simulink library "motorAndLoadSimPowerSystemsLib"  (R2019a)
settings: Solver=ode45  StartTime=0.0  StopTime=10.0  RelTol=1e-3  EnableMultiTasking=on
undefined symbols (not defined in the file): adc, encoder, inverter, pmsm, pwm
libraries: fl_lib x26, nesl_utility x16, ee_lib x6
settings Model: Creator=The MathWorks, Inc.  LastModifiedBy=The MathWorks, Inc.
settings DataIOCC: LimitDataPoints=on  SaveFormat=Array  ReturnWorkspaceOutputs=off
settings OptimizationCC: ExpressionDepthLimit=2147483647  LifeSpan=inf
settings DebuggingCC: UnderspecifiedInitializationDetection=Classic  MergeDetectMultiDrivingBlocksExec=none  SolverPrmCheckMsg=warning  AllowSymbolicDim=off  StateNameClashWarn=warning  SFUnexpectedBacktrackingDiag=warning  SFNoUnconditionalDefaultTransitionDiag=warning  SFExecutionAtInitializationDiag=none  ArithmeticOperatorsInVariantConditions=warning
settings HardwareCC: ProdBitPerPointer=32  ProdBitPerSizeT=32  ProdBitPerPtrDiffT=32  ProdLargestAtomicFloat=None  ProdIntDivRoundTo=Undefined  ProdEndianess=Unspecified  ProdWordSize=32  ProdHWDeviceType=32-bit Generic
settings ModelReferenceCC: PropagateSignalLabelsOutOfModel=off
settings SFSimCC: SimUseLocalCustomCode=off
settings RTWCC: RTWUseLocalCustomCode=off
settings CodeAppCC: StateflowObjectComments=on
settings GRTTargetCC: TargetLangStandard=C89/C90 (ANSI)  GeneratePreprocessorConditionals=Disable all
settings ConfigComp: CovMetricSettings=dw  CovHtmlReporting=on  CovSaveCumulativeToWorkspaceVar=on  CovSaveSingleToWorkspaceVar=on  CovExternalEMLEnable=off  CovSFcnEnable=off

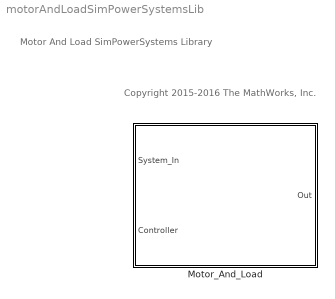
== system motorAndLoadSimPowerSystemsLib ==
  note: Motor And Load SimPowerSystems Library
  note: Copyright 2015-2016 The MathWorks, Inc.
  Motor_And_Load : Subsystem
      mask Display: image('focZynqMotorAndLoadMask.png');

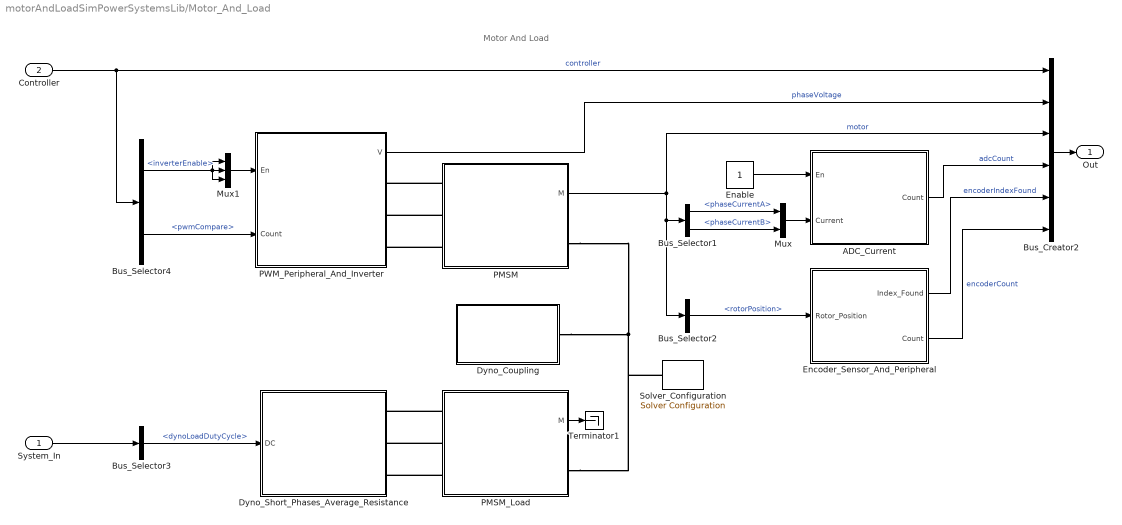
== system motorAndLoadSimPowerSystemsLib/Motor_And_Load ==
  note: Motor And Load
  System_In : Inport
  Controller : Inport  Port=2
  ADC_Current : Subsystem
      mask Display:
      | image('adcCurrentMask.png')
      | port_label('input',1,'En')
      | port_label('input',2,'I')
      | port_label('output',1,'Count')
  Bus_Creator2 : BusCreator  Inputs=6
  Bus_Selector1 : BusSelector  OutputSignals=phaseCurrentA,phaseCurrentB
  Bus_Selector2 : BusSelector  OutputSignals=rotorPosition
  Bus_Selector3 : BusSelector  OutputSignals=dynoLoadDutyCycle
  Bus_Selector4 : BusSelector  OutputSignals=inverterEnable,pwmCompare
  Dyno_Coupling : Subsystem  VariantControl=loadType == motorLoad.disc
      mask Display: image('dynoCouplingMask.png')
  Dyno_Short_Phases_Average_Resistance : Subsystem
      mask Display:
      | image('dynoShortPhasesAverageResistance.png')
      | text(0.03, 0.50, 'DC', 'HorizontalAlignment', 'Left')
      | text(0.98, 0.80, 'A',  'HorizontalAlignment', 'Right')
      | text(0.98, 0.50, 'B',  'HorizontalAlignment', 'Right')
      | text(0.98, 0.20, 'C',  'HorizontalAlignment', 'Right')
  Enable : Constant  SampleTime=-1
  Encoder_Sensor_And_Peripheral : Subsystem
      mask Display:
      | image('encoderSensorAndPeripheralMask.png')
      | port_label('input',1,'P')
      | port_label('output',1,sprintf('Index\nFound')')
      | port_label('output',2,'Count')
  Mux : Mux  Inputs=2
  Mux1 : Mux  Inputs=3
  PMSM : Subsystem
      mask Display:
      | image('pmsmMask.png')
      | text(0.03, 0.80, 'A', 'HorizontalAlignment', 'Left')
      | text(0.03, 0.50, 'B', 'HorizontalAlignment', 'Left')
      | text(0.03, 0.20, 'C', 'HorizontalAlignment', 'Left')
      | text(0.98, 0.75, 'M', 'HorizontalAlignment', 'Right')
      | text(0.98, 0.25, 'R', 'HorizontalAlignment', 'Right')
  PMSM_Load : Subsystem
      mask Display:
      | image('pmsmMask.png')
      | text(0.03, 0.80, 'A', 'HorizontalAlignment', 'Left')
      | text(0.03, 0.50, 'B', 'HorizontalAlignment', 'Left')
      | text(0.03, 0.20, 'C', 'HorizontalAlignment', 'Left')
      | text(0.98, 0.75, 'M', 'HorizontalAlignment', 'Right')
      | text(0.98, 0.25, 'R', 'HorizontalAlignment', 'Right')
  PWM_Peripheral_And_Inverter : Subsystem  VariantControl=variantPwm == enumPwm.behavior
      mask Display:
      | image('pwmPeripheralAndInverterMask.png')
      | port_label('output',1,'V')
      | port_label('input',1,'En')
      | port_label('input',2,'Compare')
      | text(0.98, 0.64, 'A', 'HorizontalAlignment', 'Right')
      | text(0.98, 0.38, 'B', 'HorizontalAlignment', 'Right')
      | text(0.98, 0.12, 'C', 'HorizontalAlignment', 'Right')
  Solver_Configuration : nesl_utility/Solver Configuration  PhysicalDomain=network_engine_domain  SubClassName=solver  LeftPortType=input  RightPortType=generic  Tones=[]  Harmonics=[]  SimulateNoise=off  Profile=off  UseLocalSampling=off  EnableSwitchedLinearOptims=on  FrequencyDomain=off  UseCCode=off  RelTol=0.001  AbsTol=1e-06  MinStep=1e-09  ToWorkspace=off  RevertToSquareIcSolve=off  NumHomotopyIterations=100  PhasorMode=off  PhasorModeNumHarmonics=1  DoDC=off  ResidualTolerance=1e-9  UseLocalSolver=on  LocalSolverChoice=NE_BACKWARD_EULER_ADVANCER  LocalSolverSampleTime=40e-6  DoFixedCost=on  MaxNonlinIter=3  MaxModeIter=2  LinearAlgebra=Sparse  EquationFormulation=NE_TIME_EF  DelaysMemoryBudget=1024  AutomaticFiltering=on  FilteringTimeConstant=0.001  PartitionStorageMethod=AS_NEEDED  PartitionMemoryBudget=1024  PartitionMethod=FAST
  Terminator1 : Terminator
  Out : Outport
  wires:
  Mux1/1 -> PWM_Peripheral_And_Inverter/1(En)
  Bus_Selector3/1 -> Dyno_Short_Phases_Average_Resistance/1(DC)  "<dynoLoadDutyCycle>"
  PMSM_Load/1(M) -> Terminator1/1
  PWM_Peripheral_And_Inverter/1(V) -> Bus_Creator2/2  "phaseVoltage"
  System_In/1 -> Bus_Selector3/1
  Encoder_Sensor_And_Peripheral/2(Count) -> Bus_Creator2/6  "encoderCount"
  Encoder_Sensor_And_Peripheral/1(Index_Found) -> Bus_Creator2/5  "encoderIndexFound"
  ADC_Current/1(Count) -> Bus_Creator2/4  "adcCount"
  Bus_Selector4/2 -> PWM_Peripheral_And_Inverter/2(Count)  "<pwmCompare>"
  Bus_Selector4/1 -> Mux1/2, Mux1/3, Mux1/1  "<inverterEnable>"
  Bus_Selector2/1 -> Encoder_Sensor_And_Peripheral/1(Rotor_Position)  "<rotorPosition>"
  Mux/1 -> ADC_Current/2(Current)
  Bus_Selector1/2 -> Mux/2  "<phaseCurrentB>"
  Bus_Selector1/1 -> Mux/1  "<phaseCurrentA>"
  Controller/1 -> Bus_Creator2/1, Bus_Selector4/1  "controller"
  Bus_Creator2/1 -> Out/1
  PMSM/1(M) -> Bus_Selector2/1, Bus_Selector1/1, Bus_Creator2/3  "motor"
  Enable/1 -> ADC_Current/1(En)
  connections:
  PMSM_Load/LConn3 -- Dyno_Short_Phases_Average_Resistance/RConn3
  PMSM_Load/LConn2 -- Dyno_Short_Phases_Average_Resistance/RConn2
  PMSM_Load/LConn1 -- Dyno_Short_Phases_Average_Resistance/RConn1
  PMSM/RConn1 -- Dyno_Coupling/RConn1 -- PMSM_Load/RConn1 -- Solver_Configuration/RConn1
  PMSM/LConn1 -- PWM_Peripheral_And_Inverter/RConn1
  PMSM/LConn2 -- PWM_Peripheral_And_Inverter/RConn2
  PMSM/LConn3 -- PWM_Peripheral_And_Inverter/RConn3

== system motorAndLoadSimPowerSystemsLib/Motor_And_Load/ADC_Current ==
  note: ADC Current
  En : Inport
  Current : Inport  Port=2
  ADC : Subsystem
      mask Display:
      | image('adcMask.png')
      | port_label('input',1,'V_T','texmode', 'on')
      | port_label('output',1,'Count')
  Current_Transducer : Subsystem
      mask Display:
      | image('currentTransducerMask.png')
      | port_label('input', 1,'En')
      | port_label('input', 2,'I')
      | port_label('output',1,'V_T','texmode', 'on')
  Count : Outport
  wires:
  Current/1 -> Current_Transducer/2(Current)
  En/1 -> Current_Transducer/1(En)
  Current_Transducer/1(V_T) -> ADC/1(Volt)  "transducerVoltage"
  ADC/1(Count) -> Count/1

== system motorAndLoadSimPowerSystemsLib/Motor_And_Load/Dyno_Coupling ==
  note: Dyno Coupling
  Inertia : fl_lib/Mechanical/Rotational Elements/Inertia  inertia=dynoCoupling.Inertia kg*m^2  w_specify=on  w_priority=High  w=pmsm.RotorVelocityInit rad/s  w_nominal_specify=off  w_nominal_unit=rad/s  w_nominal_value=1  t_specify=off  t_priority=High  t=0 N*m  t_nominal_specify=off  t_nominal_unit=N*m  t_nominal_value=1
      settings: AttributesFormatString=|
      | ---------------------------------------
      | Inertia = %<inertia>
  R : PMIOPort  Side=Right
  connections:
  Inertia/LConn1 -- R/RConn1

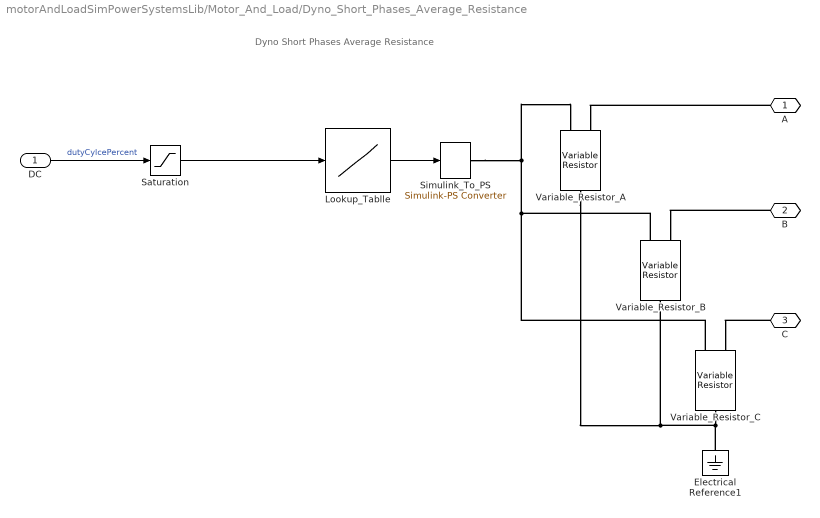
== system motorAndLoadSimPowerSystemsLib/Motor_And_Load/Dyno_Short_Phases_Average_Resistance ==
  note: Dyno Short Phases Average Resistance
  DC : Inport
  Electrical Reference1 : fl_lib/Electrical/Electrical Elements/Electrical Reference
  Lookup_Tablle : Lookup_n-D  NumberOfTableDimensions=1  BreakpointsForDimension1=[0 10 20 30 40 50 60 70 80 90 95 100]  Table=[2000 800 250 130 60 40 28 21 15 2.3 1.03 0]  ExtrapMethod=Clip  InternalRulePriority=Speed  RndMeth=Simplest  InputSameDT=on
      settings: AttributesFormatString=|
      | -----------------------------------------------------------------------
      | DutyCycle = %<BreakpointsForDimension1>
      | Resistance = %<Table>
  Saturation : Saturate  UpperLimit=100  LowerLimit=0
      settings: AttributesFormatString=|
      | ------------------------------
      | UpperLimit = %<UpperLimit>
      | LowerLimit = %<LowerLimit>
  Simulink_To_PS : nesl_utility/Simulink-PS Converter  PhysicalDomain=network_engine_domain  SubClassName=ps_input  LeftPortType=input  RightPortType=output  PseudoPeriodic=off  Frequencies=[]  NoiseDistribution=none  NoiseParameters=[]  Unit=1  AffineConversion=off  FilteringAndDerivatives=filter  SimscapeFilterOrder=1  InputFilterTimeConstant=0.001  UdotUserProvided=1
  Variable_Resistor_A : fl_lib/Electrical/Electrical Elements/Variable Resistor  Rmin=0 Ohm  i_specify=off  i_priority=None  i=0 A  i_nominal_specify=off  i_nominal_unit=A  i_nominal_value=1  v_specify=off  v_priority=None  v=0 V  v_nominal_specify=off  v_nominal_unit=V  v_nominal_value=1
  Variable_Resistor_B : fl_lib/Electrical/Electrical Elements/Variable Resistor  Rmin=0 Ohm  i_specify=off  i_priority=None  i=0 A  i_nominal_specify=off  i_nominal_unit=A  i_nominal_value=1  v_specify=off  v_priority=None  v=0 V  v_nominal_specify=off  v_nominal_unit=V  v_nominal_value=1
  Variable_Resistor_C : fl_lib/Electrical/Electrical Elements/Variable Resistor  Rmin=0 Ohm  i_specify=off  i_priority=None  i=0 A  i_nominal_specify=off  i_nominal_unit=A  i_nominal_value=1  v_specify=off  v_priority=None  v=0 V  v_nominal_specify=off  v_nominal_unit=V  v_nominal_value=1
  A : PMIOPort  Side=Right
  B : PMIOPort  Port=2  Side=Right
  C : PMIOPort  Port=3  Side=Right
  wires:
  Lookup_Tablle/1 -> Simulink_To_PS/1
  Saturation/1 -> Lookup_Tablle/1
  DC/1 -> Saturation/1  "dutyCylcePercent"
  connections:
  B/RConn1 -- Variable_Resistor_B/LConn2
  C/RConn1 -- Variable_Resistor_C/LConn2
  Variable_Resistor_C/RConn1 -- Electrical Reference1/LConn1 -- Variable_Resistor_A/RConn1 -- Variable_Resistor_B/RConn1
  A/RConn1 -- Variable_Resistor_A/LConn2
  Variable_Resistor_B/LConn1 -- Variable_Resistor_C/LConn1 -- Simulink_To_PS/RConn1 -- Variable_Resistor_A/LConn1

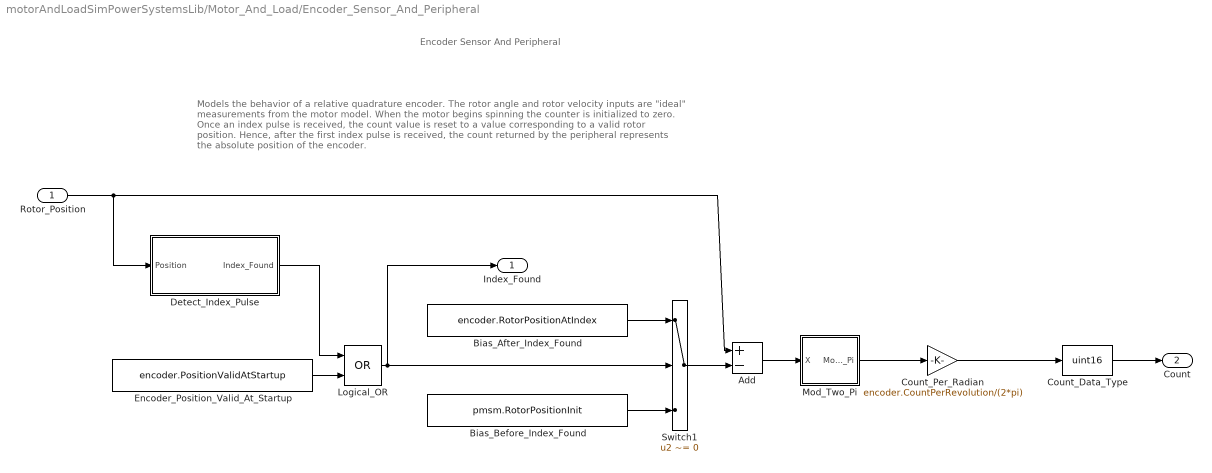
== system motorAndLoadSimPowerSystemsLib/Motor_And_Load/Encoder_Sensor_And_Peripheral ==
  note: Models the behavior of a relative quadrature encoder. The rotor angle and rotor velocity inputs are "ideal" measurements from the motor model.
      | When the motor begins spinning the counter is initialized to zero.
      | Once an index pulse is received, the count value is reset to a value corresponding to a valid rotor position.
      | Hence, after the first index pulse is received, the count returned by the peripheral represents the absolute position of the encoder.
  note: Encoder Sensor And Peripheral
  Rotor_Position : Inport
  Add : Sum  Inputs=+-
  Bias_After_Index_Found : Constant  Value=encoder.RotorPositionAtIndex
  Bias_Before_Index_Found : Constant  Value=pmsm.RotorPositionInit
  Count_Data_Type : DataTypeConversion  OutDataTypeStr=uint16
  Count_Per_Radian : Gain  Gain=encoder.CountPerRevolution/(2*pi)
      settings: AttributesFormatString=|
      | ------------------------------------------
      | Gain = %<Gain>
  Detect_Index_Pulse : Subsystem
  Encoder_Position_Valid_At_Startup : Constant  Value=encoder.PositionValidAtStartup
  Logical_OR : Logic  Operator=OR  IconShape=distinctive  AllPortsSameDT=off  OutDataTypeStr=boolean
  Mod_Two_Pi : Subsystem
      mask Display:
      | text(0.5, 0.5,'Mod 2\pi',...
      |   'HorizontalAlignment', 'Center',...
      |   'VerticalAlignment', 'Middle',...
      |   'texmode', 'on')
  Switch1 : Switch  Criteria=u2 ~= 0
  Index_Found : Outport
  Count : Outport  Port=2
  wires:
  Bias_Before_Index_Found/1 -> Switch1/3
  Bias_After_Index_Found/1 -> Switch1/1
  Logical_OR/1 -> Index_Found/1, Switch1/2
  Encoder_Position_Valid_At_Startup/1 -> Logical_OR/2
  Detect_Index_Pulse/1(Index_Found) -> Logical_OR/1
  Rotor_Position/1 -> Add/1, Detect_Index_Pulse/1(Position)
  Mod_Two_Pi/1(Mod_X_Two_Pi) -> Count_Per_Radian/1
  Count_Data_Type/1 -> Count/1
  Switch1/1 -> Add/2
  Add/1 -> Mod_Two_Pi/1(X)
  Count_Per_Radian/1 -> Count_Data_Type/1

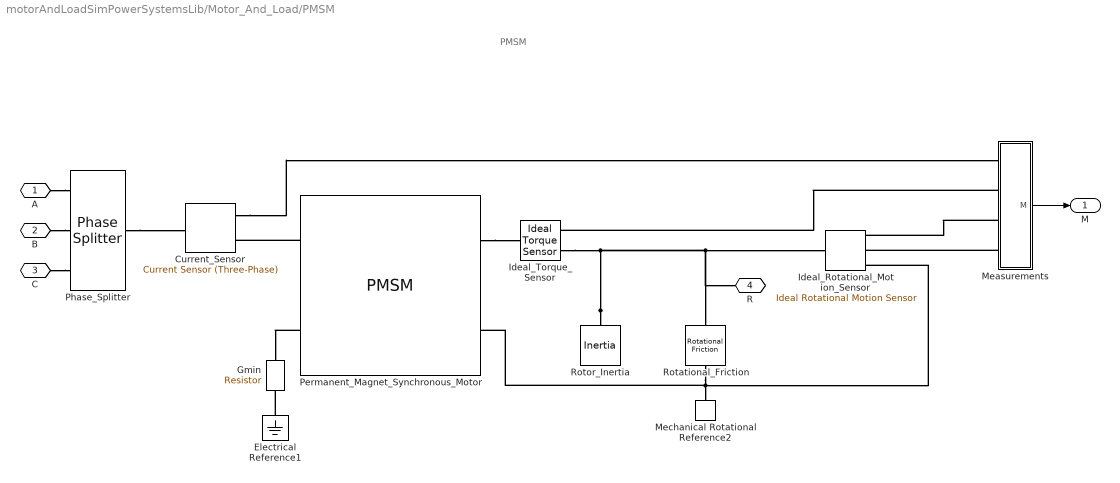
== system motorAndLoadSimPowerSystemsLib/Motor_And_Load/PMSM ==
  note: PMSM
  Current_Sensor : ee_lib/Sensors & Transducers/Current Sensor (Three-Phase)
      settings: SourceProductName=Simscape Electrical
  Electrical Reference1 : fl_lib/Electrical/Electrical Elements/Electrical Reference
  Gmin : fl_lib/Electrical/Electrical Elements/Resistor  R=1e9 Ohm  i_specify=off  i_priority=None  i=0 A  i_nominal_specify=off  i_nominal_unit=A  i_nominal_value=1  v_specify=off  v_priority=None  v=0 V  v_nominal_specify=off  v_nominal_unit=V  v_nominal_value=1
  Ideal_Rotational_Mot ion_Sensor : fl_lib/Mechanical/Mechanical Sensors/Ideal Rotational Motion Sensor  offset=pmsm.RotorPositionInit rad
  Ideal_Torque_Sensor : fl_lib/Mechanical/Mechanical Sensors/Ideal Torque Sensor
  Measurements : Subsystem
  Mechanical Rotational Reference2 : fl_lib/Mechanical/Rotational Elements/Mechanical Rotational Reference
  Permanent_Magnet_Synchronous_Motor : ee_lib/Electromechanical/Permanent Magnet/PMSM  nPolePairs=pmsm.PolePairs  pmflux_param=1  pm_flux_linkage=pmsm.FluxLinkage Wb  torque_constant=0.18 N*m/A  back_emf_constant=0.18 V/(rad/s)  stator_param=1  Ld=pmsm.InductanceLd H  Lq=pmsm.InductanceLq H  L0=pmsm.InductanceL0 H  Ls=0.0002 H  Lm=0 H  Ms=0 H  Rs=pmsm.StatorPhaseResistance Ohm  zero_sequence=ee.enum.park.zerosequence.include  J=0 kg*m^2  lam=0 N*m/(rad/s)  axes_param=2  i_d_specify=off  i_d_priority=None  i_d=0 A  i_d_nominal_specify=off  i_d_nominal_unit=A  i_d_nominal_value=1  i_q_specify=off  i_q_priority=None  i_q=0 A  i_q_nominal_specify=off  i_q_nominal_unit=A  i_q_nominal_value=1  torque_specify=off  torque_priority=None  torque=0 N*m  torque_nominal_specify=off  torque_nominal_unit=N*m  torque_nominal_value=1  angular_velocity_specify=on  angular_velocity_priority=None  angular_velocity=0 rpm  angular_velocity_nominal_specify=off  angular_velocity_nominal_unit=rpm  angular_velocity_nominal_value=1  angular_position_specify=on  angular_position_priority=High  angular_position=pmsm.RotorPositionInit rad  angular_position_nominal_specify=off  angular_position_nominal_unit=deg  angular_position_nominal_value=1
      settings: SourceProductName=Simscape Electrical
  Phase_Splitter : ee_lib/Connectors & References/Phase Splitter
      settings: SourceProductName=Simscape Electrical  SourceProductBaseCode=PS
  Rotational_Friction : fl_lib/Mechanical/Rotational Elements/Rotational Friction  brkwy_trq=pmsm.BreakawayFrictionTorque N*m  brkwy_vel=0.060623 rad/s  Col_trq=pmsm.CoulombFrictionTorque N*m  visc_coef=pmsm.ViscousFrictionCoefficient N*m/(rad/s)  w_specify=off  w_priority=None  w=0 rad/s  w_nominal_specify=off  w_nominal_unit=rad/s  w_nominal_value=1  t_specify=off  t_priority=None  t=0 N*m  t_nominal_specify=off  t_nominal_unit=N*m  t_nominal_value=1
      settings: SourceProductName=Simscape
  Rotor_Inertia : fl_lib/Mechanical/Rotational Elements/Inertia  inertia=pmsm.Inertia kg*m^2  w_specify=on  w_priority=High  w=pmsm.RotorVelocityInit rad/s  w_nominal_specify=off  w_nominal_unit=rad/s  w_nominal_value=1  t_specify=off  t_priority=None  t=0 N*m  t_nominal_specify=off  t_nominal_unit=N*m  t_nominal_value=1
  A : PMIOPort  Side=Left
  B : PMIOPort  Port=2  Side=Left
  C : PMIOPort  Port=3  Side=Left
  R : PMIOPort  Port=4  Side=Right
  M : Outport
  wires:
  Measurements/1(M) -> M/1
  connections:
  Measurements/LConn4 -- Ideal_Rotational_Mot ion_Sensor/RConn2
  Measurements/LConn3 -- Ideal_Rotational_Mot ion_Sensor/RConn3
  Measurements/LConn2 -- Ideal_Torque_Sensor/RConn2
  Permanent_Magnet_Synchronous_Motor/LConn1 -- Current_Sensor/RConn2
  C/RConn1 -- Phase_Splitter/RConn3
  B/RConn1 -- Phase_Splitter/RConn2
  A/RConn1 -- Phase_Splitter/RConn1
  Permanent_Magnet_Synchronous_Motor/LConn2 -- Gmin/RConn1
  Mechanical Rotational Reference2/LConn1 -- Permanent_Magnet_Synchronous_Motor/RConn2 -- Ideal_Rotational_Mot ion_Sensor/RConn1 -- Rotational_Friction/RConn1
  Phase_Splitter/LConn1 -- Current_Sensor/LConn1
  Current_Sensor/RConn1 -- Measurements/LConn1
  Electrical Reference1/LConn1 -- Gmin/LConn1
  Permanent_Magnet_Synchronous_Motor/RConn1 -- Ideal_Torque_Sensor/LConn1
  Rotor_Inertia/LConn1 -- Ideal_Rotational_Mot ion_Sensor/LConn1 -- Rotational_Friction/LConn1 -- R/RConn1 -- Ideal_Torque_Sensor/RConn1

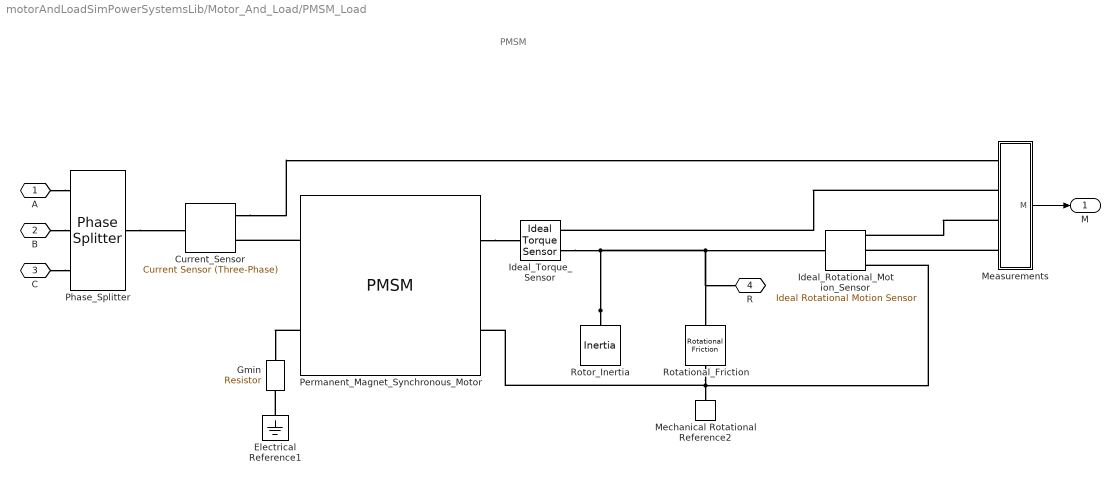
== system motorAndLoadSimPowerSystemsLib/Motor_And_Load/PMSM_Load ==
  note: PMSM
  Current_Sensor : ee_lib/Sensors & Transducers/Current Sensor (Three-Phase)
      settings: SourceProductName=Simscape Electrical
  Electrical Reference1 : fl_lib/Electrical/Electrical Elements/Electrical Reference
  Gmin : fl_lib/Electrical/Electrical Elements/Resistor  R=1e9 Ohm  i_specify=off  i_priority=None  i=0 A  i_nominal_specify=off  i_nominal_unit=A  i_nominal_value=1  v_specify=off  v_priority=None  v=0 V  v_nominal_specify=off  v_nominal_unit=V  v_nominal_value=1
  Ideal_Rotational_Mot ion_Sensor : fl_lib/Mechanical/Mechanical Sensors/Ideal Rotational Motion Sensor  offset=pmsm.RotorPositionInit rad
  Ideal_Torque_Sensor : fl_lib/Mechanical/Mechanical Sensors/Ideal Torque Sensor
  Measurements : Subsystem
  Mechanical Rotational Reference2 : fl_lib/Mechanical/Rotational Elements/Mechanical Rotational Reference
  Permanent_Magnet_Synchronous_Motor : ee_lib/Electromechanical/Permanent Magnet/PMSM  nPolePairs=pmsm.PolePairs  pmflux_param=1  pm_flux_linkage=pmsm.FluxLinkage Wb  torque_constant=0.18 N*m/A  back_emf_constant=0.18 V/(rad/s)  stator_param=1  Ld=pmsm.InductanceLd H  Lq=pmsm.InductanceLq H  L0=pmsm.InductanceL0 H  Ls=0.0002 H  Lm=0 H  Ms=0 H  Rs=pmsm.StatorPhaseResistance Ohm  zero_sequence=ee.enum.park.zerosequence.include  J=0 kg*m^2  lam=0 N*m/(rad/s)  axes_param=2  i_d_specify=off  i_d_priority=None  i_d=0 A  i_d_nominal_specify=off  i_d_nominal_unit=A  i_d_nominal_value=1  i_q_specify=off  i_q_priority=None  i_q=0 A  i_q_nominal_specify=off  i_q_nominal_unit=A  i_q_nominal_value=1  torque_specify=off  torque_priority=None  torque=0 N*m  torque_nominal_specify=off  torque_nominal_unit=N*m  torque_nominal_value=1  angular_velocity_specify=on  angular_velocity_priority=None  angular_velocity=0 rpm  angular_velocity_nominal_specify=off  angular_velocity_nominal_unit=rpm  angular_velocity_nominal_value=1  angular_position_specify=on  angular_position_priority=High  angular_position=pmsm.RotorPositionInit rad  angular_position_nominal_specify=off  angular_position_nominal_unit=deg  angular_position_nominal_value=1
      settings: SourceProductName=Simscape Electrical
  Phase_Splitter : ee_lib/Connectors & References/Phase Splitter
      settings: SourceProductName=Simscape Electrical  SourceProductBaseCode=PS
  Rotational_Friction : fl_lib/Mechanical/Rotational Elements/Rotational Friction  brkwy_trq=pmsm.BreakawayFrictionTorque N*m  brkwy_vel=0.060623 rad/s  Col_trq=pmsm.CoulombFrictionTorque N*m  visc_coef=pmsm.ViscousFrictionCoefficient N*m/(rad/s)  w_specify=off  w_priority=None  w=0 rad/s  w_nominal_specify=off  w_nominal_unit=rad/s  w_nominal_value=1  t_specify=off  t_priority=None  t=0 N*m  t_nominal_specify=off  t_nominal_unit=N*m  t_nominal_value=1
      settings: SourceProductName=Simscape
  Rotor_Inertia : fl_lib/Mechanical/Rotational Elements/Inertia  inertia=pmsm.Inertia kg*m^2  w_specify=on  w_priority=High  w=pmsm.RotorVelocityInit rad/s  w_nominal_specify=off  w_nominal_unit=rad/s  w_nominal_value=1  t_specify=off  t_priority=None  t=0 N*m  t_nominal_specify=off  t_nominal_unit=N*m  t_nominal_value=1
  A : PMIOPort  Side=Left
  B : PMIOPort  Port=2  Side=Left
  C : PMIOPort  Port=3  Side=Left
  R : PMIOPort  Port=4  Side=Right
  M : Outport
  wires:
  Measurements/1(M) -> M/1
  connections:
  Measurements/LConn4 -- Ideal_Rotational_Mot ion_Sensor/RConn2
  Measurements/LConn3 -- Ideal_Rotational_Mot ion_Sensor/RConn3
  Measurements/LConn2 -- Ideal_Torque_Sensor/RConn2
  Permanent_Magnet_Synchronous_Motor/LConn1 -- Current_Sensor/RConn2
  C/RConn1 -- Phase_Splitter/RConn3
  B/RConn1 -- Phase_Splitter/RConn2
  A/RConn1 -- Phase_Splitter/RConn1
  Permanent_Magnet_Synchronous_Motor/LConn2 -- Gmin/RConn1
  Mechanical Rotational Reference2/LConn1 -- Permanent_Magnet_Synchronous_Motor/RConn2 -- Ideal_Rotational_Mot ion_Sensor/RConn1 -- Rotational_Friction/RConn1
  Phase_Splitter/LConn1 -- Current_Sensor/LConn1
  Current_Sensor/RConn1 -- Measurements/LConn1
  Electrical Reference1/LConn1 -- Gmin/LConn1
  Permanent_Magnet_Synchronous_Motor/RConn1 -- Ideal_Torque_Sensor/LConn1
  Rotor_Inertia/LConn1 -- Ideal_Rotational_Mot ion_Sensor/LConn1 -- Rotational_Friction/LConn1 -- R/RConn1 -- Ideal_Torque_Sensor/RConn1

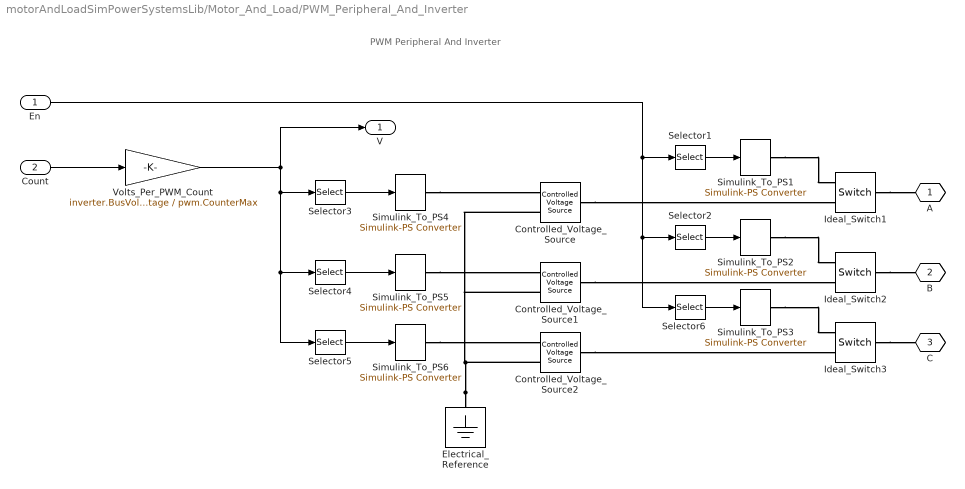
== system motorAndLoadSimPowerSystemsLib/Motor_And_Load/PWM_Peripheral_And_Inverter ==
  note: PWM Peripheral And Inverter
  En : Inport
  Count : Inport  Port=2
  Controlled_Voltage_Source : fl_lib/Electrical/Electrical Sources/Controlled Voltage Source
  Controlled_Voltage_Source1 : fl_lib/Electrical/Electrical Sources/Controlled Voltage Source
  Controlled_Voltage_Source2 : fl_lib/Electrical/Electrical Sources/Controlled Voltage Source
  Electrical_Reference : fl_lib/Electrical/Electrical Elements/Electrical Reference
  Ideal_Switch1 : fl_lib/Electrical/Electrical Elements/Switch  R_closed=0.0001 Ohm  G_open=1e-5 1/Ohm  Threshold=0  i_specify=off  i_priority=None  i=0 A  i_nominal_specify=off  i_nominal_unit=A  i_nominal_value=1  v_specify=off  v_priority=None  v=0 V  v_nominal_specify=off  v_nominal_unit=V  v_nominal_value=1
      settings: SourceProductName=Simscape
  Ideal_Switch2 : fl_lib/Electrical/Electrical Elements/Switch  R_closed=0.0001 Ohm  G_open=1e-5 1/Ohm  Threshold=0  i_specify=off  i_priority=None  i=0 A  i_nominal_specify=off  i_nominal_unit=A  i_nominal_value=1  v_specify=off  v_priority=None  v=0 V  v_nominal_specify=off  v_nominal_unit=V  v_nominal_value=1
      settings: SourceProductName=Simscape
  Ideal_Switch3 : fl_lib/Electrical/Electrical Elements/Switch  R_closed=0.0001 Ohm  G_open=1e-5 1/Ohm  Threshold=0  i_specify=off  i_priority=None  i=0 A  i_nominal_specify=off  i_nominal_unit=A  i_nominal_value=1  v_specify=off  v_priority=None  v=0 V  v_nominal_specify=off  v_nominal_unit=V  v_nominal_value=1
      settings: SourceProductName=Simscape
  Selector1 : Selector  InputPortWidth=3  IndexOptions=Index vector (dialog)  Indices=[1]  OutputSizes=1
  Selector2 : Selector  InputPortWidth=3  IndexOptions=Index vector (dialog)  Indices=2  OutputSizes=1
  Selector3 : Selector  InputPortWidth=3  IndexOptions=Index vector (dialog)  Indices=[1]  OutputSizes=1
  Selector4 : Selector  InputPortWidth=3  IndexOptions=Index vector (dialog)  Indices=2  OutputSizes=1
  Selector5 : Selector  InputPortWidth=3  IndexOptions=Index vector (dialog)  Indices=3  OutputSizes=1
  Selector6 : Selector  InputPortWidth=3  IndexOptions=Index vector (dialog)  Indices=3  OutputSizes=1
  Simulink_To_PS{1..6} (6 alike) : nesl_utility/Simulink-PS Converter  PhysicalDomain=network_engine_domain  SubClassName=ps_input  LeftPortType=input  RightPortType=output  PseudoPeriodic=off  Frequencies=[]  NoiseDistribution=none  NoiseParameters=[]  Unit=1  AffineConversion=off  FilteringAndDerivatives=zero  SimscapeFilterOrder=1  InputFilterTimeConstant=0.001  UdotUserProvided=1
  Volts_Per_PWM_Count : Gain  Gain=inverter.BusVoltage / pwm.CounterMax  ParamDataTypeStr=double  OutDataTypeStr=double
      settings: AttributesFormatString=|
      | ----------------------------------------------------------------
      | Gain = %<Gain>
  A : PMIOPort  Tag=PMCPort  Side=Right
  B : PMIOPort  Tag=PMCPort  Port=2  Side=Right
  C : PMIOPort  Tag=PMCPort  Port=3  Side=Right
  V : Outport
  wires:
  Selector6/1 -> Simulink_To_PS3/1
  Selector2/1 -> Simulink_To_PS2/1
  Count/1 -> Volts_Per_PWM_Count/1
  En/1 -> Selector1/1, Selector6/1, Selector2/1
  Volts_Per_PWM_Count/1 -> Selector4/1, Selector5/1, Selector3/1, V/1
  Selector5/1 -> Simulink_To_PS6/1
  Selector4/1 -> Simulink_To_PS5/1
  Selector3/1 -> Simulink_To_PS4/1
  Selector1/1 -> Simulink_To_PS1/1
  connections:
  Electrical_Reference/LConn1 -- Controlled_Voltage_Source1/RConn2 -- Controlled_Voltage_Source/RConn2 -- Controlled_Voltage_Source2/RConn2
  Simulink_To_PS5/RConn1 -- Controlled_Voltage_Source1/RConn1
  Simulink_To_PS6/RConn1 -- Controlled_Voltage_Source2/RConn1
  Controlled_Voltage_Source2/LConn1 -- Ideal_Switch3/RConn2
  Controlled_Voltage_Source1/LConn1 -- Ideal_Switch2/RConn2
  Controlled_Voltage_Source/LConn1 -- Ideal_Switch1/RConn2
  Simulink_To_PS4/RConn1 -- Controlled_Voltage_Source/RConn1
  Simulink_To_PS3/RConn1 -- Ideal_Switch3/RConn1
  Simulink_To_PS2/RConn1 -- Ideal_Switch2/RConn1
  Simulink_To_PS1/RConn1 -- Ideal_Switch1/RConn1
  Ideal_Switch3/LConn1 -- C/RConn1
  Ideal_Switch2/LConn1 -- B/RConn1
  Ideal_Switch1/LConn1 -- A/RConn1

== system motorAndLoadSimPowerSystemsLib/Motor_And_Load/ADC_Current/ADC ==
  note: ADC
  Volt : Inport
  Add : Sum
  Count_At_Zero_Transducer_Volt : Constant  Value=adc.CountAtZeroTransducerVolt  SampleTime=-1
  Count_Per_Transducer_Volt : Constant  Value=adc.CountPerTransducerVolt
  Data_Type_Conversion : DataTypeConversion  OutDataTypeStr=adc.DataType  SaturateOnIntegerOverflow=on
      settings: AttributesFormatString=------------------------\nDT = %<OutDataTypeStr>
  Product : Product  RndMeth=Zero
  Saturation : Saturate  UpperLimit=adc.CountMax  LowerLimit=adc.CountMin
      settings: AttributesFormatString=|
      | ----------------------------
      | Upper = %<UpperLimit>
      | Lower = %<LowerLimit>
  Transport_Delay : TransportDelay  DelayTime=adc.Delay
      settings: AttributesFormatString=-----------------------------\nDelay = %<DelayTime>
  Count : Outport
  wires:
  Transport_Delay/1 -> Product/1
  Saturation/1 -> Data_Type_Conversion/1
  Count_Per_Transducer_Volt/1 -> Product/2
  Data_Type_Conversion/1 -> Count/1
  Volt/1 -> Transport_Delay/1
  Product/1 -> Add/1
  Add/1 -> Saturation/1
  Count_At_Zero_Transducer_Volt/1 -> Add/2

== system motorAndLoadSimPowerSystemsLib/Motor_And_Load/ADC_Current/Current_Transducer ==
  note: Current Transducer
  En : Inport
  Current : Inport  Port=2
  ADC_Transducer_Volt_At_Zero_Ampere : Constant  Value=adc.TransducerVoltAtZeroAmpere
  ADC_Transducer_Volt_Per_Ampere : Constant  Value=adc.TransducerVoltPerAmpere
  Add : Sum
  Product : Product  RndMeth=Zero
  Switch : Switch  Criteria=u2 ~= 0
  Zero : Constant  Value=0
  V_T : Outport
  wires:
  ADC_Transducer_Volt_At_Zero_Ampere/1 -> Add/2
  Product/1 -> Add/1
  ADC_Transducer_Volt_Per_Ampere/1 -> Product/2
  Current/1 -> Product/1
  Zero/1 -> Switch/3  "disabled"
  Switch/1 -> V_T/1  "transducerVoltage"
  Add/1 -> Switch/1  "enabled"
  En/1 -> Switch/2  "enableTransducer"

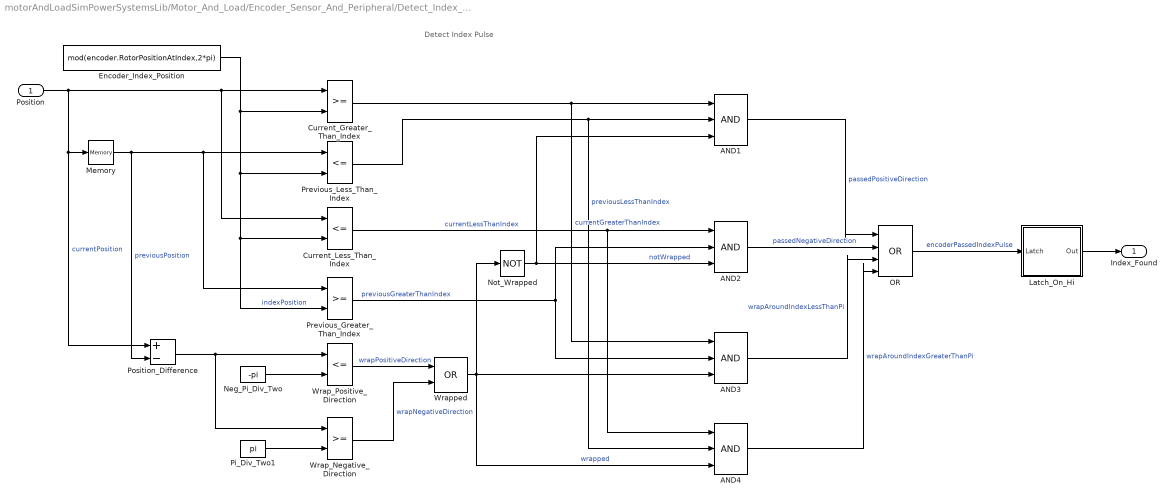
== system motorAndLoadSimPowerSystemsLib/Motor_And_Load/Encoder_Sensor_And_Peripheral/Detect_Index_Pulse ==
  note: Detect Index Pulse
  Position : Inport
  AND{1..4} (4 alike) : Logic  Inputs=3  IconShape=distinctive  AllPortsSameDT=off  OutDataTypeStr=boolean
  Current_Greater_Than_Index : RelationalOperator  OutDataTypeStr=boolean  RndMeth=Nearest
  Current_Less_Than_Index : RelationalOperator  Operator=<=  OutDataTypeStr=boolean  RndMeth=Nearest
  Encoder_Index_Position : Constant  Value=mod(encoder.RotorPositionAtIndex,2*pi)  SampleTime=-1
  Latch_On_Hi : Subsystem
  Memory : Memory
  Neg_Pi_Div_Two : Constant  Value=-pi
  Not_Wrapped : Logic  Operator=NOT  IconShape=distinctive  AllPortsSameDT=off  OutDataTypeStr=boolean
  OR : Logic  Operator=OR  Inputs=4  IconShape=distinctive  AllPortsSameDT=off  OutDataTypeStr=boolean
  Pi_Div_Two1 : Constant  Value=pi
  Position_Difference : Sum  Inputs=+-
  Previous_Greater_Than_Index : RelationalOperator  OutDataTypeStr=boolean  RndMeth=Nearest
  Previous_Less_Than_Index : RelationalOperator  Operator=<=  OutDataTypeStr=boolean  RndMeth=Nearest
  Wrap_Negative_Direction : RelationalOperator  OutDataTypeStr=boolean  RndMeth=Nearest
  Wrap_Positive_Direction : RelationalOperator  Operator=<=  OutDataTypeStr=boolean  RndMeth=Nearest
  Wrapped : Logic  Operator=OR  IconShape=distinctive  AllPortsSameDT=off  OutDataTypeStr=boolean
  Index_Found : Outport
  wires:
  AND2/1 -> OR/2  "passedNegativeDirection"
  AND1/1 -> OR/1  "passedPositiveDirection"
  Current_Less_Than_Index/1 -> AND2/1, AND4/1  "currentLessThanIndex"
  Previous_Greater_Than_Index/1 -> AND2/2, AND3/2  "previousGreaterThanIndex"
  OR/1 -> Latch_On_Hi/1(Latch)  "encoderPassedIndexPulse"
  Encoder_Index_Position/1 -> Previous_Less_Than_Index/2, Previous_Greater_Than_Index/2, Current_Less_Than_Index/2, Current_Greater_Than_Index/2  "indexPosition"
  Previous_Less_Than_Index/1 -> AND1/2, AND4/2  "previousLessThanIndex"
  Current_Greater_Than_Index/1 -> AND3/1, AND1/1  "currentGreaterThanIndex"
  Memory/1 -> Position_Difference/2, Previous_Greater_Than_Index/1, Previous_Less_Than_Index/1  "previousPosition"
  Position/1 -> Position_Difference/1, Memory/1, Current_Less_Than_Index/1, Current_Greater_Than_Index/1  "currentPosition"
  Position_Difference/1 -> Wrap_Negative_Direction/1, Wrap_Positive_Direction/1
  Wrap_Positive_Direction/1 -> Wrapped/1  "wrapPositiveDirection"
  Neg_Pi_Div_Two/1 -> Wrap_Positive_Direction/2
  Wrap_Negative_Direction/1 -> Wrapped/2  "wrapNegativeDirection"
  Pi_Div_Two1/1 -> Wrap_Negative_Direction/2
  AND3/1 -> OR/3  "wrapAroundIndexLessThanPi"
  Latch_On_Hi/1(Out) -> Index_Found/1
  Not_Wrapped/1 -> AND1/3, AND2/3  "notWrapped"
  Wrapped/1 -> AND4/3, AND3/3, Not_Wrapped/1  "wrapped"
  AND4/1 -> OR/4  "wrapAroundIndexGreaterThanPi"

== system motorAndLoadSimPowerSystemsLib/Motor_And_Load/Encoder_Sensor_And_Peripheral/Mod_Two_Pi ==
  note: Mod Two Pi
  X : Inport
  Mod : Math  Operator=mod  SaturateOnIntegerOverflow=on
  Two_Pi : Constant  Value=2*pi  OutDataTypeStr=Inherit: Inherit via back propagation
  Mod_X_Two_Pi : Outport
  wires:
  X/1 -> Mod/1
  Two_Pi/1 -> Mod/2
  Mod/1 -> Mod_X_Two_Pi/1

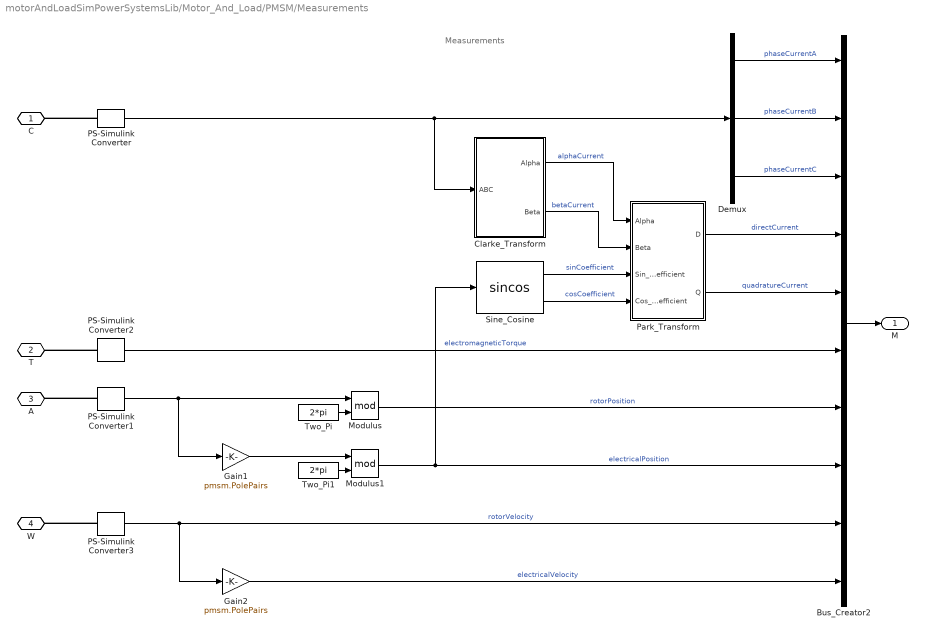
== system motorAndLoadSimPowerSystemsLib/Motor_And_Load/PMSM/Measurements ==
  note: Measurements
  Bus_Creator2 : BusCreator  Inputs=10
  Clarke_Transform : Subsystem
      mask Display:
      | port_label('input',1,'ABC')
      | port_label('output',1,'\alpha','texmode', 'on')
      | port_label('output',2,'\beta','texmode', 'on')
  Demux : Demux  Outputs=3
  Gain1 : Gain  Gain=pmsm.PolePairs
      settings: AttributesFormatString=-----------------------------\n%<Gain>
  Gain2 : Gain  Gain=pmsm.PolePairs
      settings: AttributesFormatString=-----------------------------\n%<Gain>
  Modulus : Math  Operator=mod  SaturateOnIntegerOverflow=on
  Modulus1 : Math  Operator=mod  SaturateOnIntegerOverflow=on
  PS-Simulink Converter : nesl_utility/PS-Simulink Converter  PhysicalDomain=network_engine_domain  SubClassName=ps_output  LeftPortType=input  RightPortType=output  PseudoPeriodic=off  Frequencies=[]  Unit=A  AffineConversion=off
  PS-Simulink Converter1 : nesl_utility/PS-Simulink Converter  PhysicalDomain=network_engine_domain  SubClassName=ps_output  LeftPortType=input  RightPortType=output  PseudoPeriodic=off  Frequencies=[]  Unit=rad  AffineConversion=off
  PS-Simulink Converter2 : nesl_utility/PS-Simulink Converter  PhysicalDomain=network_engine_domain  SubClassName=ps_output  LeftPortType=input  RightPortType=output  PseudoPeriodic=off  Frequencies=[]  Unit=N*m  AffineConversion=off
  PS-Simulink Converter3 : nesl_utility/PS-Simulink Converter  PhysicalDomain=network_engine_domain  SubClassName=ps_output  LeftPortType=input  RightPortType=output  PseudoPeriodic=off  Frequencies=[]  Unit=rad/s  AffineConversion=off
  Park_Transform : Subsystem
      mask Display:
      | port_label('input',1,'\alpha','texmode', 'on')
      | port_label('input',2,'\beta','texmode', 'on')
      | port_label('input',3,'Sin')
      | port_label('input',4,'Cos')
      | port_label('output',1,'D')
      | port_label('output',2,'Q')
  Sine_Cosine : Trigonometry  Operator=sincos
  Two_Pi : Constant  Value=2*pi  OutDataTypeStr=Inherit: Inherit via back propagation
  Two_Pi1 : Constant  Value=2*pi  OutDataTypeStr=Inherit: Inherit via back propagation
  C : PMIOPort  Side=Left
  T : PMIOPort  Port=2  Side=Left
  A : PMIOPort  Port=3  Side=Left
  W : PMIOPort  Port=4  Side=Left
  M : Outport
  wires:
  Demux/2 -> Bus_Creator2/2  "phaseCurrentB"
  Demux/3 -> Bus_Creator2/3  "phaseCurrentC"
  Demux/1 -> Bus_Creator2/1  "phaseCurrentA"
  PS-Simulink Converter/1 -> Clarke_Transform/1(ABC), Demux/1
  Bus_Creator2/1 -> M/1
  PS-Simulink Converter2/1 -> Bus_Creator2/6  "electromagneticTorque"
  PS-Simulink Converter3/1 -> Bus_Creator2/9, Gain2/1  "rotorVelocity"
  Modulus/1 -> Bus_Creator2/7  "rotorPosition"
  Modulus1/1 -> Sine_Cosine/1, Bus_Creator2/8  "electricalPosition"
  Gain2/1 -> Bus_Creator2/10  "electricalVelocity"
  Two_Pi/1 -> Modulus/2
  Two_Pi1/1 -> Modulus1/2
  Gain1/1 -> Modulus1/1
  PS-Simulink Converter1/1 -> Modulus/1, Gain1/1
  Sine_Cosine/1 -> Park_Transform/3(Sin_Coefficient)  "sinCoefficient"
  Sine_Cosine/2 -> Park_Transform/4(Cos_Coefficient)  "cosCoefficient"
  Clarke_Transform/2(Beta) -> Park_Transform/2(Beta)  "betaCurrent"
  Clarke_Transform/1(Alpha) -> Park_Transform/1(Alpha)  "alphaCurrent"
  Park_Transform/1(D) -> Bus_Creator2/4  "directCurrent"
  Park_Transform/2(Q) -> Bus_Creator2/5  "quadratureCurrent"
  connections:
  PS-Simulink Converter/LConn1 -- C/RConn1
  PS-Simulink Converter1/LConn1 -- A/RConn1
  PS-Simulink Converter2/LConn1 -- T/RConn1
  PS-Simulink Converter3/LConn1 -- W/RConn1

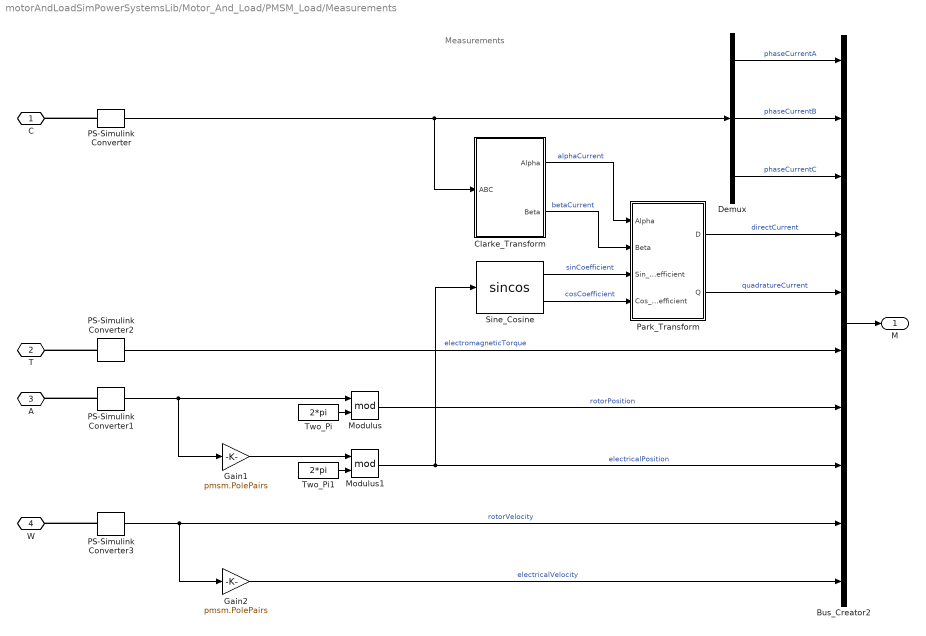
== system motorAndLoadSimPowerSystemsLib/Motor_And_Load/PMSM_Load/Measurements ==
  note: Measurements
  Bus_Creator2 : BusCreator  Inputs=10
  Clarke_Transform : Subsystem
      mask Display:
      | port_label('input',1,'ABC')
      | port_label('output',1,'\alpha','texmode', 'on')
      | port_label('output',2,'\beta','texmode', 'on')
  Demux : Demux  Outputs=3
  Gain1 : Gain  Gain=pmsm.PolePairs
      settings: AttributesFormatString=-----------------------------\n%<Gain>
  Gain2 : Gain  Gain=pmsm.PolePairs
      settings: AttributesFormatString=-----------------------------\n%<Gain>
  Modulus : Math  Operator=mod  SaturateOnIntegerOverflow=on
  Modulus1 : Math  Operator=mod  SaturateOnIntegerOverflow=on
  PS-Simulink Converter : nesl_utility/PS-Simulink Converter  PhysicalDomain=network_engine_domain  SubClassName=ps_output  LeftPortType=input  RightPortType=output  PseudoPeriodic=off  Frequencies=[]  Unit=A  AffineConversion=off
  PS-Simulink Converter1 : nesl_utility/PS-Simulink Converter  PhysicalDomain=network_engine_domain  SubClassName=ps_output  LeftPortType=input  RightPortType=output  PseudoPeriodic=off  Frequencies=[]  Unit=rad  AffineConversion=off
  PS-Simulink Converter2 : nesl_utility/PS-Simulink Converter  PhysicalDomain=network_engine_domain  SubClassName=ps_output  LeftPortType=input  RightPortType=output  PseudoPeriodic=off  Frequencies=[]  Unit=N*m  AffineConversion=off
  PS-Simulink Converter3 : nesl_utility/PS-Simulink Converter  PhysicalDomain=network_engine_domain  SubClassName=ps_output  LeftPortType=input  RightPortType=output  PseudoPeriodic=off  Frequencies=[]  Unit=rad/s  AffineConversion=off
  Park_Transform : Subsystem
      mask Display:
      | port_label('input',1,'\alpha','texmode', 'on')
      | port_label('input',2,'\beta','texmode', 'on')
      | port_label('input',3,'Sin')
      | port_label('input',4,'Cos')
      | port_label('output',1,'D')
      | port_label('output',2,'Q')
  Sine_Cosine : Trigonometry  Operator=sincos
  Two_Pi : Constant  Value=2*pi  OutDataTypeStr=Inherit: Inherit via back propagation
  Two_Pi1 : Constant  Value=2*pi  OutDataTypeStr=Inherit: Inherit via back propagation
  C : PMIOPort  Side=Left
  T : PMIOPort  Port=2  Side=Left
  A : PMIOPort  Port=3  Side=Left
  W : PMIOPort  Port=4  Side=Left
  M : Outport
  wires:
  Demux/2 -> Bus_Creator2/2  "phaseCurrentB"
  Demux/3 -> Bus_Creator2/3  "phaseCurrentC"
  Demux/1 -> Bus_Creator2/1  "phaseCurrentA"
  PS-Simulink Converter/1 -> Clarke_Transform/1(ABC), Demux/1
  Bus_Creator2/1 -> M/1
  PS-Simulink Converter2/1 -> Bus_Creator2/6  "electromagneticTorque"
  PS-Simulink Converter3/1 -> Bus_Creator2/9, Gain2/1  "rotorVelocity"
  Modulus/1 -> Bus_Creator2/7  "rotorPosition"
  Modulus1/1 -> Sine_Cosine/1, Bus_Creator2/8  "electricalPosition"
  Gain2/1 -> Bus_Creator2/10  "electricalVelocity"
  Two_Pi/1 -> Modulus/2
  Two_Pi1/1 -> Modulus1/2
  Gain1/1 -> Modulus1/1
  PS-Simulink Converter1/1 -> Modulus/1, Gain1/1
  Sine_Cosine/1 -> Park_Transform/3(Sin_Coefficient)  "sinCoefficient"
  Sine_Cosine/2 -> Park_Transform/4(Cos_Coefficient)  "cosCoefficient"
  Clarke_Transform/2(Beta) -> Park_Transform/2(Beta)  "betaCurrent"
  Clarke_Transform/1(Alpha) -> Park_Transform/1(Alpha)  "alphaCurrent"
  Park_Transform/1(D) -> Bus_Creator2/4  "directCurrent"
  Park_Transform/2(Q) -> Bus_Creator2/5  "quadratureCurrent"
  connections:
  PS-Simulink Converter/LConn1 -- C/RConn1
  PS-Simulink Converter1/LConn1 -- A/RConn1
  PS-Simulink Converter2/LConn1 -- T/RConn1
  PS-Simulink Converter3/LConn1 -- W/RConn1

== system motorAndLoadSimPowerSystemsLib/Motor_And_Load/Encoder_Sensor_And_Peripheral/Detect_Index_Pulse/Latch_On_Hi ==
  note: Latch On Hi
  Latch : Inport
  IC : InitialCondition  Value=0
  Memory : Memory
  One : Constant  OutDataTypeStr=boolean
  Switch : Switch  Criteria=u2 ~= 0  Threshold=1
  Out : Outport
  wires:
  IC/1 -> Memory/1, Out/1
  Latch/1 -> Switch/3
  Switch/1 -> IC/1
  One/1 -> Switch/1
  Memory/1 -> Switch/2

== system motorAndLoadSimPowerSystemsLib/Motor_And_Load/PMSM/Measurements/Clarke_Transform ==
  note: Clarke Transform
  ABC : Inport
  A : Selector  IndexMode=Zero-based  InputPortWidth=3  IndexOptions=Index vector (dialog)  Indices=0  OutputSizes=1
  Add : Sum  OutDataTypeStr=Inherit: Same as first input
  Alpha_Gain : Gain  Gain=1/sqrt(3)
  B : Selector  IndexMode=Zero-based  InputPortWidth=3  IndexOptions=Index vector (dialog)  Indices=1  OutputSizes=1
  Beta_Gain : Gain  Gain=2/sqrt(3)
  Alpha : Outport
  Beta : Outport  Port=2
  wires:
  Add/1 -> Beta/1
  B/1 -> Beta_Gain/1
  Beta_Gain/1 -> Add/2
  ABC/1 -> A/1, B/1
  Alpha_Gain/1 -> Add/1
  A/1 -> Alpha_Gain/1, Alpha/1

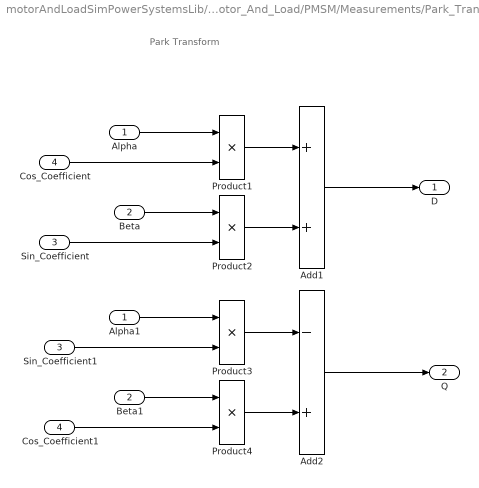
== system motorAndLoadSimPowerSystemsLib/Motor_And_Load/PMSM/Measurements/Park_Transform ==
  note: Park Transform
  Alpha : Inport
  Beta : Inport  Port=2
  Sin_Coefficient : Inport  Port=3
  Cos_Coefficient : Inport  Port=4
  Add1 : Sum  OutDataTypeStr=Inherit: Same as first input
  Add2 : Sum  Inputs=-+  OutDataTypeStr=Inherit: Same as first input
  Alpha1 : InportShadow
  Beta1 : InportShadow  Port=2
  Cos_Coefficient1 : InportShadow  Port=4
  Product{1..4} (4 alike) : Product  RndMeth=Simplest
  Sin_Coefficient1 : InportShadow  Port=3
  D : Outport
  Q : Outport  Port=2
  wires:
  Product3/1 -> Add2/1
  Product4/1 -> Add2/2
  Product1/1 -> Add1/1
  Product2/1 -> Add1/2
  Alpha1/1 -> Product3/1
  Sin_Coefficient1/1 -> Product3/2
  Cos_Coefficient1/1 -> Product4/2
  Beta1/1 -> Product4/1
  Alpha/1 -> Product1/1
  Cos_Coefficient/1 -> Product1/2
  Beta/1 -> Product2/1
  Sin_Coefficient/1 -> Product2/2
  Add1/1 -> D/1
  Add2/1 -> Q/1

== system motorAndLoadSimPowerSystemsLib/Motor_And_Load/PMSM_Load/Measurements/Clarke_Transform ==
  note: Clarke Transform
  ABC : Inport
  A : Selector  IndexMode=Zero-based  InputPortWidth=3  IndexOptions=Index vector (dialog)  Indices=0  OutputSizes=1
  Add : Sum  OutDataTypeStr=Inherit: Same as first input
  Alpha_Gain : Gain  Gain=1/sqrt(3)
  B : Selector  IndexMode=Zero-based  InputPortWidth=3  IndexOptions=Index vector (dialog)  Indices=1  OutputSizes=1
  Beta_Gain : Gain  Gain=2/sqrt(3)
  Alpha : Outport
  Beta : Outport  Port=2
  wires:
  Add/1 -> Beta/1
  B/1 -> Beta_Gain/1
  Beta_Gain/1 -> Add/2
  ABC/1 -> A/1, B/1
  Alpha_Gain/1 -> Add/1
  A/1 -> Alpha_Gain/1, Alpha/1

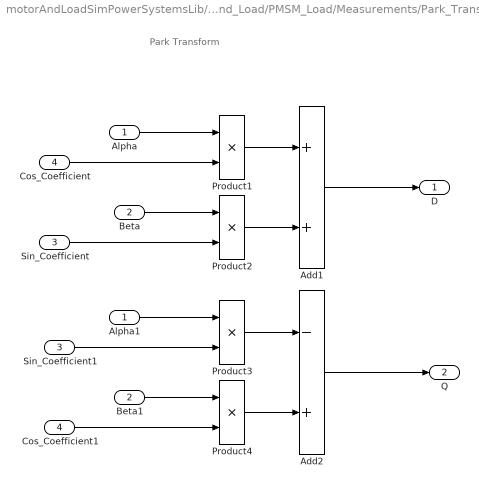
== system motorAndLoadSimPowerSystemsLib/Motor_And_Load/PMSM_Load/Measurements/Park_Transform ==
  note: Park Transform
  Alpha : Inport
  Beta : Inport  Port=2
  Sin_Coefficient : Inport  Port=3
  Cos_Coefficient : Inport  Port=4
  Add1 : Sum  OutDataTypeStr=Inherit: Same as first input
  Add2 : Sum  Inputs=-+  OutDataTypeStr=Inherit: Same as first input
  Alpha1 : InportShadow
  Beta1 : InportShadow  Port=2
  Cos_Coefficient1 : InportShadow  Port=4
  Product{1..4} (4 alike) : Product  RndMeth=Simplest
  Sin_Coefficient1 : InportShadow  Port=3
  D : Outport
  Q : Outport  Port=2
  wires:
  Product3/1 -> Add2/1
  Product4/1 -> Add2/2
  Product1/1 -> Add1/1
  Product2/1 -> Add1/2
  Alpha1/1 -> Product3/1
  Sin_Coefficient1/1 -> Product3/2
  Cos_Coefficient1/1 -> Product4/2
  Beta1/1 -> Product4/1
  Alpha/1 -> Product1/1
  Cos_Coefficient/1 -> Product1/2
  Beta/1 -> Product2/1
  Sin_Coefficient/1 -> Product2/2
  Add1/1 -> D/1
  Add2/1 -> Q/1
